simulink model "Reference"  (R2025b)
settings: Solver=FixedStepAuto  StartTime=0.0  StopTime=1  FixedStep=1e-3  RelTol=1e-3
undefined symbols (not defined in the file or in its folder): cfg
settings Model: Creator=nikol  LastModifiedBy=nikol

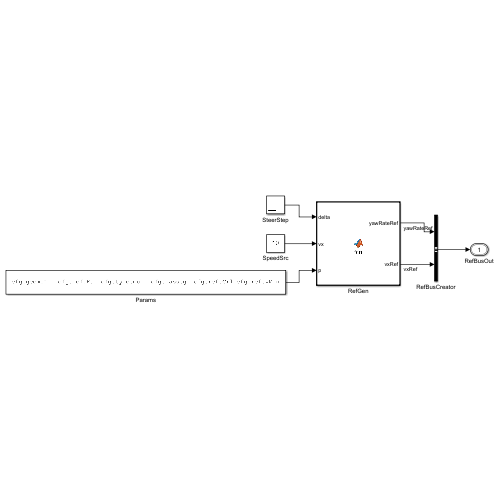
[thumbnail: Simulink's stored preview of the top-level diagram]
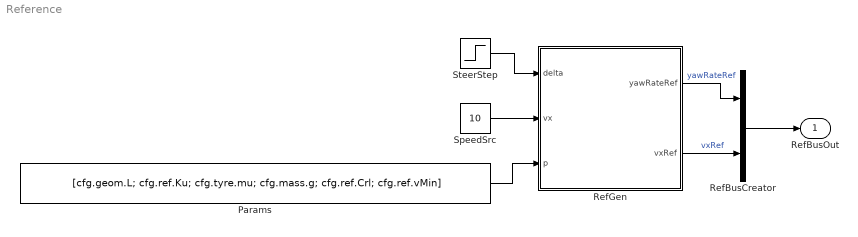
== system Reference ==
  Params : Constant  Value=[cfg.geom.L; cfg.ref.Ku; cfg.tyre.mu; cfg.mass.g; cfg.ref.Crl; cfg.ref.vMin]
  RefBusCreator : BusCreator  Inputs=2  OutDataTypeStr=Bus: RefBus
  RefGen : MATLAB Function  TreatAsAtomicUnit=on
  SpeedSrc : Constant  Value=10
  SteerStep : Step  After=0.05  SampleTime=0
  RefBusOut : Outport  OutDataTypeStr=Bus: RefBus
  wires:
  SteerStep/1 -> RefGen/1(delta)
  SpeedSrc/1 -> RefGen/2(vx)
  RefGen/1(yawRateRef) -> RefBusCreator/1  "yawRateRef"
  Params/1 -> RefGen/3(p)
  RefGen/2(vxRef) -> RefBusCreator/2  "vxRef"
  RefBusCreator/1 -> RefBusOut/1

== matlab function Reference/RefGen ==
  data: delta input; yawRateRef output; vx input; p input; vxRef output
function [yawRateRef, vxRef] = fcn(delta, vx, p)
    [yawRateRef, vxRef] = referenceGen(delta, vx, p);
end
